simulink model "model_1heater"  (R2023b)
settings: Solver=VariableStepAuto  StartTime=0.0  StopTime=2000  RelTol=1e-3
values from neighbouring files (symbols this model uses):
  C2K = 273.15    [dual_heater1.m]    (also in dual_heater_linear.m; one_heater1.m; variables.m)
  K1 = (U*A)/(m*cp)    (= 0.0035)    [dual_heater1.m]    (also in dual_heater_linear.m; one_heater1.m = 0.006)
  K2 = (eps*sig*A)/(m*cp)    (= 9.9225e-12)    [dual_heater1.m]    (also in dual_heater_linear.m; one_heater1.m = 1.701e-11)
  K3 = (U*As)/(m*cp)    (= 0.0025)    [dual_heater1.m]    (also in dual_heater_linear.m)
  K4 = (eps*sig*As)/(m*cp)    (= 7.0875e-12)    [dual_heater1.m]    (also in dual_heater_linear.m)
  Ku1 = alfa/(m*cp)    (= 0.005)    [dual_heater1.m]    (also in dual_heater_linear.m; one_heater1.m)
  T0 = T0 + C2K    (= 296.15)    [dual_heater1.m]    (also in dual_heater_linear.m; one_heater1.m)
  T_inf = T_inf + C2K    (= 296.15)    [dual_heater1.m]    (also in dual_heater_linear.m; one_heater1.m; variables.m)
settings Model: Creator=Ondra  LastModifiedBy=Ondra

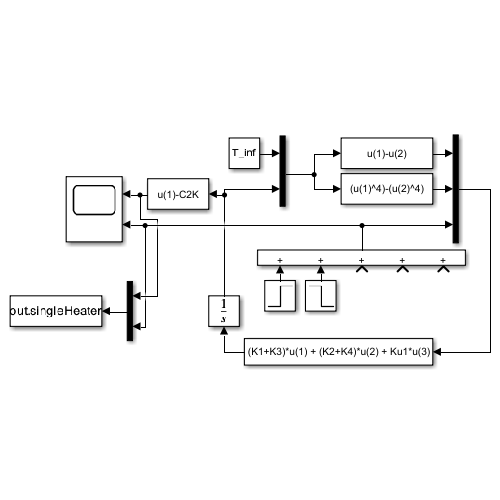
[thumbnail: Simulink's stored preview of the top-level diagram]
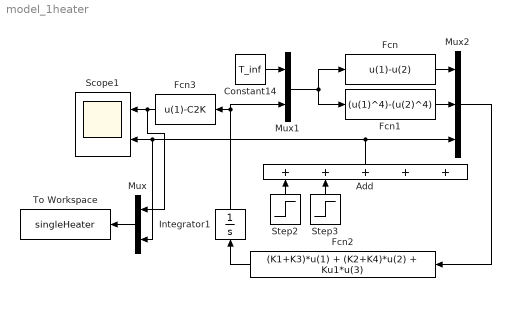
== system model_1heater ==
  Add : Sum  Inputs=+++++
  Constant14 : Constant  Value=T_inf
  Fcn : Fcn  Expr=u(1)-u(2)
  Fcn1 : Fcn  Expr=(u(1)^4)-(u(2)^4)
  Fcn2 : Fcn  Expr=(K1+K3)*u(1) + (K2+K4)*u(2) + Ku1*u(3)
  Fcn3 : Fcn  Expr=u(1)-C2K
  Integrator1 : Integrator  InitialCondition=T0
  Mux : Mux  Inputs=2
  Mux1 : Mux  Inputs=2
  Mux2 : Mux  Inputs=3
  Scope1 : Scope  NumInputPorts=2
  Step2 : Step  After=50  SampleTime=0
  Step3 : Step  Time=1000  After=-50  SampleTime=0
  To Workspace : ToWorkspace  VariableName=singleHeater  SaveFormat=Timeseries  SampleTime=-1
  wires:
  Constant14/1 -> Mux1/1
  Integrator1/1 -> Fcn3/1, Mux1/2
  Mux1/1 -> Fcn1/1, Fcn/1
  Fcn/1 -> Mux2/1
  Fcn1/1 -> Mux2/2
  Mux2/1 -> Fcn2/1
  Fcn2/1 -> Integrator1/1
  Step2/1 -> Add/1
  Step3/1 -> Add/2
  Add/1 -> Mux/2, Scope1/2, Mux2/3
  Fcn3/1 -> Mux/1, Scope1/1
  Mux/1 -> To Workspace/1
